simulink model "gm_IP_Core_SS_Switch_and_PWM"  (R2018a)
settings: Solver=VariableStepAuto  StartTime=0.0  StopTime=0.05  RelTol=1e-3
undefined symbols (not defined in the file or in its folder): T_pwm_clk
libraries: hdlmdlgenlib x5, hdlsllib x1
settings Model: Creator=BHK  LastModifiedBy=Wendel
settings OptimizationCC: BlockReduction=off  ConditionallyExecuteInputs=off  DefaultParameterBehavior=Inlined
settings DebuggingCC: AlgebraicLoopMsg=error  InheritedTsInSrcMsg=none
settings HardwareCC: ProdBitPerPointer=32  ProdBitPerSizeT=32  ProdBitPerPtrDiffT=32  ProdLargestAtomicFloat=None  ProdIntDivRoundTo=Undefined  ProdEndianess=Unspecified  ProdWordSize=32  ProdHWDeviceType=ASIC/FPGA->ASIC/FPGA  TargetBitPerPointer=64  TargetBitPerSizeT=64  TargetBitPerPtrDiffT=64  TargetLongLongMode=on  TargetIntDivRoundTo=Zero  TargetEndianess=LittleEndian  TargetWordSize=64  TargetHWDeviceType=Custom Processor->MATLAB Host Computer  ProdEqTarget=off

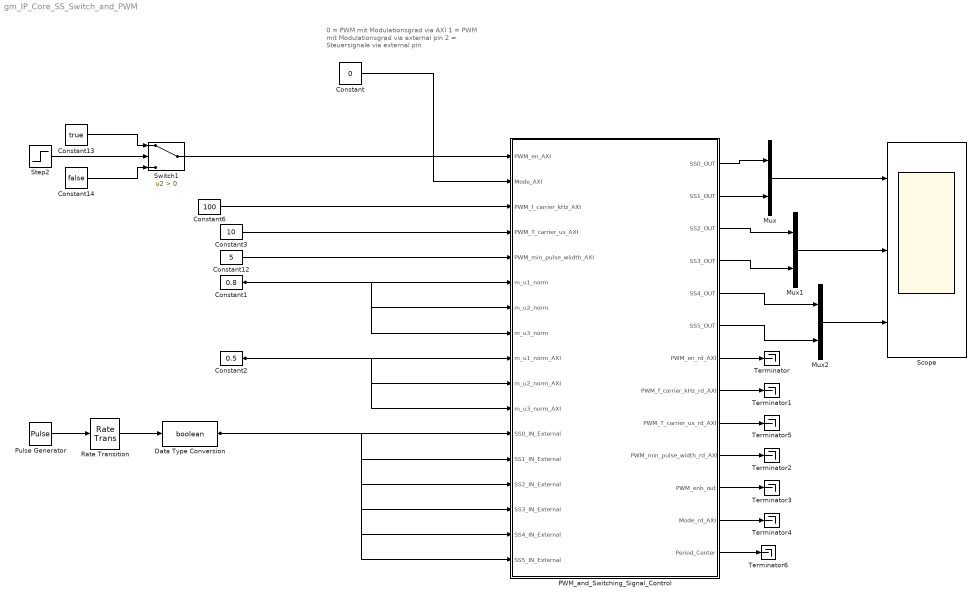
== system gm_IP_Core_SS_Switch_and_PWM ==
  note: 0 = PWM mit Modulationsgrad via AXI
      | 1 = PWM mit Modulationsgrad via external pin
      | 2 = Steuersignale via external pin
  Constant : Constant  Value=0  OutDataTypeStr=fixdt(0,2,0)  SampleTime=T_pwm_clk
  Constant1 : Constant  Value=0.8  OutDataTypeStr=fixdt(1,14,12)  SampleTime=T_pwm_clk
  Constant12 : Constant  Value=5  OutDataTypeStr=fixdt(0,8,0)  SampleTime=T_pwm_clk
  Constant13 : Constant  Value=true  SampleTime=T_pwm_clk
  Constant14 : Constant  Value=false  SampleTime=T_pwm_clk
  Constant2 : Constant  Value=0.5  OutDataTypeStr=fixdt(1,14,12)  SampleTime=T_pwm_clk
  Constant3 : Constant  Value=10  OutDataTypeStr=fixdt(0,8,0)  SampleTime=T_pwm_clk
  Constant6 : Constant  Value=100  OutDataTypeStr=fixdt(0,8,0)  SampleTime=T_pwm_clk
  Data Type Conversion : DataTypeConversion  OutDataTypeStr=boolean
  Mux : Mux  Inputs=2
  Mux1 : Mux  Inputs=2
  Mux2 : Mux  Inputs=2
  PWM_and_Switching_Signal_Control : Subsystem  TreatAsAtomicUnit=on
  Pulse Generator : DiscretePulseGenerator  PulseType=Time based  Period=0.01  PulseWidth=5
  Rate Transition : RateTransition  OutPortSampleTime=T_pwm_clk
  Scope : Scope  NumInputPorts=3
  Step2 : Step  Time=0.002  SampleTime=T_pwm_clk
  Switch1 : Switch  Criteria=u2 > Threshold
  Terminator{,1..6} (7 alike) : Terminator
  wires:
  PWM_and_Switching_Signal_Control/13(Period_Center) -> Terminator6/1
  PWM_and_Switching_Signal_Control/9(PWM_T_carrier_us_rd_AXI) -> Terminator5/1
  Pulse Generator/1 -> Rate Transition/1
  Rate Transition/1 -> Data Type Conversion/1
  Constant3/1 -> PWM_and_Switching_Signal_Control/4(PWM_T_carrier_us_AXI)
  Data Type Conversion/1 -> PWM_and_Switching_Signal_Control/12(SS0_IN_External), PWM_and_Switching_Signal_Control/14(SS2_IN_External), PWM_and_Switching_Signal_Control/16(SS4_IN_External), PWM_and_Switching_Signal_Control/13(SS1_IN_External), PWM_and_Switching_Signal_Control/15(SS3_IN_External), PWM_and_Switching_Signal_Control/17(SS5_IN_External)
  Mux1/1 -> Scope/2
  Mux2/1 -> Scope/3
  PWM_and_Switching_Signal_Control/6(SS5_OUT) -> Mux2/2
  PWM_and_Switching_Signal_Control/5(SS4_OUT) -> Mux2/1
  PWM_and_Switching_Signal_Control/4(SS3_OUT) -> Mux1/2
  PWM_and_Switching_Signal_Control/3(SS2_OUT) -> Mux1/1
  Mux/1 -> Scope/1
  PWM_and_Switching_Signal_Control/2(SS1_OUT) -> Mux/2
  PWM_and_Switching_Signal_Control/1(SS0_OUT) -> Mux/1
  Constant2/1 -> PWM_and_Switching_Signal_Control/11(m_u3_norm_AXI), PWM_and_Switching_Signal_Control/10(m_u2_norm_AXI), PWM_and_Switching_Signal_Control/9(m_u1_norm_AXI)
  PWM_and_Switching_Signal_Control/12(Mode_rd_AXI) -> Terminator4/1
  PWM_and_Switching_Signal_Control/11(PWM_enb_out) -> Terminator3/1
  PWM_and_Switching_Signal_Control/10(PWM_min_pulse_width_rd_AXI) -> Terminator2/1
  PWM_and_Switching_Signal_Control/8(PWM_f_carrier_kHz_rd_AXI) -> Terminator1/1
  PWM_and_Switching_Signal_Control/7(PWM_en_rd_AXI) -> Terminator/1
  Constant1/1 -> PWM_and_Switching_Signal_Control/7(m_u2_norm), PWM_and_Switching_Signal_Control/8(m_u3_norm), PWM_and_Switching_Signal_Control/6(m_u1_norm)
  Constant12/1 -> PWM_and_Switching_Signal_Control/5(PWM_min_pulse_wiidth_AXI)
  Constant6/1 -> PWM_and_Switching_Signal_Control/3(PWM_f_carrier_kHz_AXI)
  Constant/1 -> PWM_and_Switching_Signal_Control/2(Mode_AXI)
  Switch1/1 -> PWM_and_Switching_Signal_Control/1(PWM_en_AXI)
  Constant14/1 -> Switch1/3
  Constant13/1 -> Switch1/1
  Step2/1 -> Switch1/2

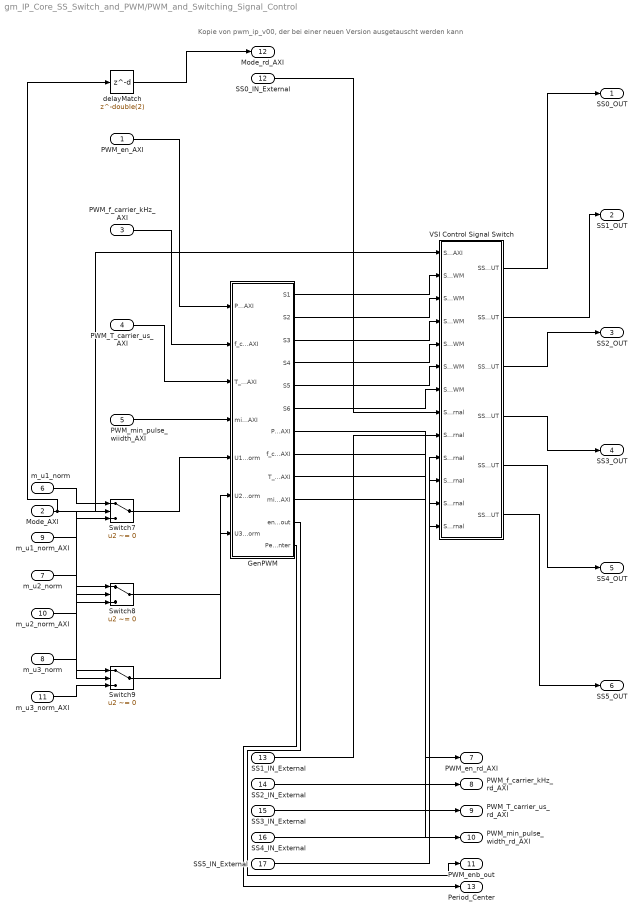
== system gm_IP_Core_SS_Switch_and_PWM/PWM_and_Switching_Signal_Control ==
  note: Kopie von pwm_ip_v00, der bei einer neuen Version ausgetauscht werden kann
  PWM_en_AXI : Inport  OutDataTypeStr=boolean  PortDimensions=1  SampleTime=1e-08
  Mode_AXI : Inport  Port=2  OutDataTypeStr=fixdt(0, 2, 0)  PortDimensions=1  SampleTime=1e-08
  PWM_f_carrier_kHz_AXI : Inport  Port=3  OutDataTypeStr=uint8  PortDimensions=1  SampleTime=1e-08
  PWM_T_carrier_us_AXI : Inport  Port=4  OutDataTypeStr=uint8  PortDimensions=1  SampleTime=1e-08
  PWM_min_pulse_wiidth_AXI : Inport  Port=5  OutDataTypeStr=uint8  PortDimensions=1  SampleTime=1e-08
  m_u1_norm : Inport  Port=6  OutDataTypeStr=fixdt(1, 14, 12)  PortDimensions=1  SampleTime=1e-08
  m_u2_norm : Inport  Port=7  OutDataTypeStr=fixdt(1, 14, 12)  PortDimensions=1  SampleTime=1e-08
  m_u3_norm : Inport  Port=8  OutDataTypeStr=fixdt(1, 14, 12)  PortDimensions=1  SampleTime=1e-08
  m_u1_norm_AXI : Inport  Port=9  OutDataTypeStr=fixdt(1, 14, 12)  PortDimensions=1  SampleTime=1e-08
  m_u2_norm_AXI : Inport  Port=10  OutDataTypeStr=fixdt(1, 14, 12)  PortDimensions=1  SampleTime=1e-08
  m_u3_norm_AXI : Inport  Port=11  OutDataTypeStr=fixdt(1, 14, 12)  PortDimensions=1  SampleTime=1e-08
  SS0_IN_External : Inport  Port=12  OutDataTypeStr=boolean  PortDimensions=1  SampleTime=1e-08
  SS1_IN_External : Inport  Port=13  OutDataTypeStr=boolean  PortDimensions=1  SampleTime=1e-08
  SS2_IN_External : Inport  Port=14  OutDataTypeStr=boolean  PortDimensions=1  SampleTime=1e-08
  SS3_IN_External : Inport  Port=15  OutDataTypeStr=boolean  PortDimensions=1  SampleTime=1e-08
  SS4_IN_External : Inport  Port=16  OutDataTypeStr=boolean  PortDimensions=1  SampleTime=1e-08
  SS5_IN_External : Inport  Port=17  OutDataTypeStr=boolean  PortDimensions=1  SampleTime=1e-08
  GenPWM : Subsystem
  Switch7 : Switch  Criteria=u2 ~= 0  Threshold=double(0)  OutDataTypeStr=fixdt(1, 14, 12)  SampleTime=1e-08
  Switch8 : Switch  Criteria=u2 ~= 0  Threshold=double(0)  OutDataTypeStr=fixdt(1, 14, 12)  SampleTime=1e-08
  Switch9 : Switch  Criteria=u2 ~= 0  Threshold=double(0)  OutDataTypeStr=fixdt(1, 14, 12)  SampleTime=1e-08
  VSI Control Signal Switch : Subsystem
  delayMatch : Delay  DelayLength=double(2)  InitialCondition=0  InputProcessing=Inherited  SampleTime=1e-08
  SS0_OUT : Outport
  SS1_OUT : Outport  Port=2
  SS2_OUT : Outport  Port=3
  SS3_OUT : Outport  Port=4
  SS4_OUT : Outport  Port=5
  SS5_OUT : Outport  Port=6
  PWM_en_rd_AXI : Outport  Port=7
  PWM_f_carrier_kHz_rd_AXI : Outport  Port=8
  PWM_T_carrier_us_rd_AXI : Outport  Port=9
  PWM_min_pulse_width_rd_AXI : Outport  Port=10
  PWM_enb_out : Outport  Port=11
  Mode_rd_AXI : Outport  Port=12
  Period_Center : Outport  Port=13
  wires:
  PWM_en_AXI/1 -> GenPWM/1(PWM_en_AXI)
  delayMatch/1 -> Mode_rd_AXI/1
  PWM_f_carrier_kHz_AXI/1 -> GenPWM/2(f_carrier_kHz_AXI)
  PWM_T_carrier_us_AXI/1 -> GenPWM/3(T_carrier_us_AXI)
  PWM_min_pulse_wiidth_AXI/1 -> GenPWM/4(min_pulse_width_AXI)
  m_u1_norm/1 -> Switch7/1
  m_u2_norm/1 -> Switch8/1
  m_u3_norm/1 -> Switch9/1
  m_u1_norm_AXI/1 -> Switch7/3
  m_u2_norm_AXI/1 -> Switch8/3
  m_u3_norm_AXI/1 -> Switch9/3
  SS0_IN_External/1 -> VSI Control Signal Switch/8(SS0_IN_External)
  SS1_IN_External/1 -> VSI Control Signal Switch/9(SS1_IN_External)
  SS2_IN_External/1 -> VSI Control Signal Switch/10(SS2_IN_External)
  SS3_IN_External/1 -> VSI Control Signal Switch/11(SS3_IN_External)
  SS4_IN_External/1 -> VSI Control Signal Switch/12(SS4_IN_External)
  SS5_IN_External/1 -> VSI Control Signal Switch/13(SS5_IN_External)
  GenPWM/1(S1) -> VSI Control Signal Switch/2(SS0_IN_PWM)
  GenPWM/2(S2) -> VSI Control Signal Switch/3(SS1_IN_PWM)
  GenPWM/3(S3) -> VSI Control Signal Switch/4(SS2_IN_PWM)
  GenPWM/4(S4) -> VSI Control Signal Switch/5(SS3_IN_PWM)
  GenPWM/5(S5) -> VSI Control Signal Switch/6(SS4_IN_PWM)
  GenPWM/6(S6) -> VSI Control Signal Switch/7(SS5_IN_PWM)
  GenPWM/7(PWM_en_rd_AXI) -> PWM_en_rd_AXI/1
  GenPWM/8(f_carrier_kHz_rd_AXI) -> PWM_f_carrier_kHz_rd_AXI/1
  GenPWM/9(T_carrier_us_rd_AXI) -> PWM_T_carrier_us_rd_AXI/1
  GenPWM/10(min_pulse_width_rd_AXI) -> PWM_min_pulse_width_rd_AXI/1
  GenPWM/11(enb_out) -> PWM_enb_out/1
  GenPWM/12(Period_Center) -> Period_Center/1
  Switch7/1 -> GenPWM/5(U1_norm)
  Switch8/1 -> GenPWM/6(U2_norm)
  Switch9/1 -> GenPWM/7(U3_norm)
  VSI Control Signal Switch/1(SS0_OUT) -> SS0_OUT/1
  VSI Control Signal Switch/2(SS1_OUT) -> SS1_OUT/1
  VSI Control Signal Switch/3(SS2_OUT) -> SS2_OUT/1
  VSI Control Signal Switch/4(SS3_OUT) -> SS3_OUT/1
  VSI Control Signal Switch/5(SS4_OUT) -> SS4_OUT/1
  VSI Control Signal Switch/6(SS5_OUT) -> SS5_OUT/1
  Mode_AXI/1 -> delayMatch/1, Switch9/2, Switch8/2, Switch7/2, VSI Control Signal Switch/1(Switch_AXI)

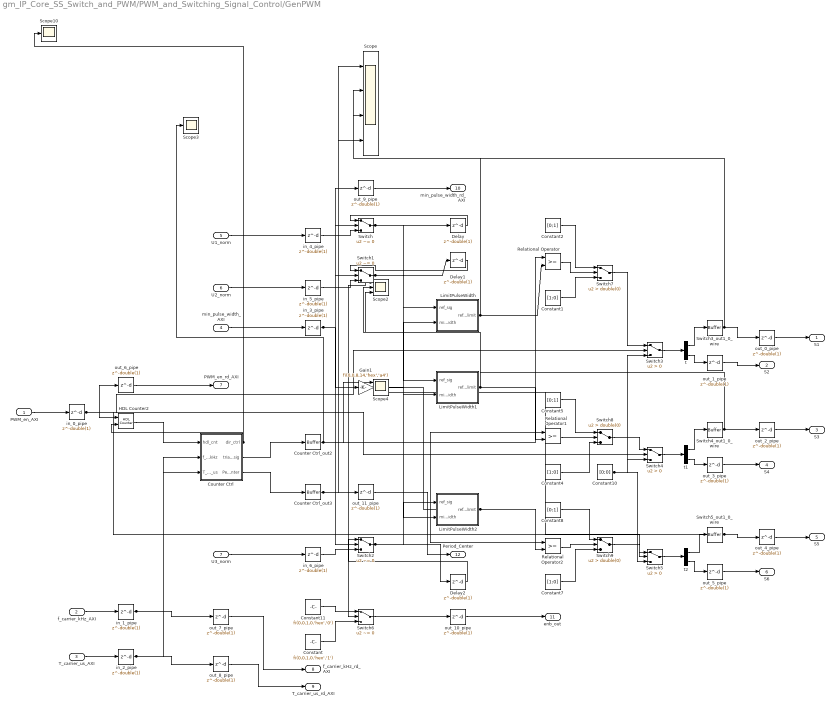
== system gm_IP_Core_SS_Switch_and_PWM/PWM_and_Switching_Signal_Control/GenPWM ==
  PWM_en_AXI : Inport  PortDimensions=1  SampleTime=1e-08
  f_carrier_kHz_AXI : Inport  Port=2  PortDimensions=1  SampleTime=1e-08
  T_carrier_us_AXI : Inport  Port=3  PortDimensions=1  SampleTime=1e-08
  min_pulse_width_AXI : Inport  Port=4  PortDimensions=1  SampleTime=1e-08
  U1_norm : Inport  Port=5  PortDimensions=1  SampleTime=1e-08
  U2_norm : Inport  Port=6  PortDimensions=1  SampleTime=1e-08
  U3_norm : Inport  Port=7  PortDimensions=1  SampleTime=1e-08
  Constant : Constant  Value=fi(0,0,1,0,'hex','1')  OutDataTypeStr=boolean  SampleTime=-1
  Constant1 : Constant  Value=[1;0]  OutDataTypeStr=fixdt(0, 1, 0)  SampleTime=-1
  Constant10 : Constant  Value=[0;0]  OutDataTypeStr=fixdt(0, 1, 0)  SampleTime=-1
  Constant11 : Constant  Value=fi(0,0,1,0,'hex','0')  OutDataTypeStr=boolean  SampleTime=-1
  Constant2 : Constant  Value=[0;1]  OutDataTypeStr=fixdt(0, 1, 0)  SampleTime=-1
  Constant4 : Constant  Value=[1;0]  OutDataTypeStr=fixdt(0, 1, 0)  SampleTime=-1
  Constant5 : Constant  Value=[0;1]  OutDataTypeStr=fixdt(0, 1, 0)  SampleTime=-1
  Constant7 : Constant  Value=[1;0]  OutDataTypeStr=fixdt(0, 1, 0)  SampleTime=-1
  Constant8 : Constant  Value=[0;1]  OutDataTypeStr=fixdt(0, 1, 0)  SampleTime=-1
  Counter Ctrl : Subsystem
  Counter Ctrl_out2 : hdlmdlgenlib/Buffer
      settings: SourceProductName=HDL Coder  SourceProductBaseCode=HD
  Counter Ctrl_out3 : hdlmdlgenlib/Buffer
      settings: SourceProductName=HDL Coder  SourceProductBaseCode=HD
  Delay : Delay  DelayLength=double(1)  InitialCondition=0  InputProcessing=Inherited  SampleTime=1e-08
  Delay1 : Delay  DelayLength=double(1)  InitialCondition=0  InputProcessing=Inherited  SampleTime=1e-08
  Delay2 : Delay  DelayLength=double(1)  InitialCondition=0  InputProcessing=Inherited  SampleTime=1e-08
  Gain1 : Gain  Gain=fi(0,0,8,14,'hex','a4')  ParamDataTypeStr=fixdt(0, 8, 14)  OutDataTypeStr=fixdt(1, 18, 10)  SampleTime=1e-08
  HDL Counter2 : hdlsllib/Sources/HDL Counter  CountType=Free running  CountInit=double(0)  CountStep=double(1)  CountMax=25  CountFromType=Initial value  CountFrom=double(0)  CountResetPort=off  CountLoadPort=off  CountEnbPort=on  CountDirPort=on  CountDataType=Unsigned  CountWordLen=20  CountFracLen=0  CountSampTime=1e-08
      settings: SourceProductBaseCode=HD
  LimitPulseWidth : Subsystem
  LimitPulseWidth1 : Subsystem
  LimitPulseWidth2 : Subsystem
  Relational Operator : RelationalOperator  OutDataTypeStr=boolean  SampleTime=1e-08  RndMeth=Nearest
  Relational Operator1 : RelationalOperator  OutDataTypeStr=boolean  SampleTime=1e-08  RndMeth=Nearest
  Relational Operator2 : RelationalOperator  OutDataTypeStr=boolean  SampleTime=1e-08  RndMeth=Nearest
  Scope : Scope  NumInputPorts=4
  Scope10 : Scope
  Scope2 : Scope  NumInputPorts=3
  Scope3 : Scope
  Scope4 : Scope  NumInputPorts=3
  Switch : Switch  Criteria=u2 ~= 0  Threshold=double(0)  OutDataTypeStr=fixdt(1, 14, 12)  SampleTime=1e-08
  Switch1 : Switch  Criteria=u2 ~= 0  Threshold=double(0)  OutDataTypeStr=fixdt(1, 14, 12)  SampleTime=1e-08
  Switch2 : Switch  Criteria=u2 ~= 0  Threshold=double(0)  OutDataTypeStr=fixdt(1, 14, 12)  SampleTime=1e-08
  Switch3 : Switch  Criteria=u2 > Threshold  OutDataTypeStr=fixdt(0, 1, 0)  SampleTime=1e-08
  Switch3_out1_0_wire : hdlmdlgenlib/Buffer
      settings: SourceProductName=HDL Coder  SourceProductBaseCode=HD
  Switch4 : Switch  Criteria=u2 > Threshold  OutDataTypeStr=fixdt(0, 1, 0)  SampleTime=1e-08
  Switch4_out1_0_wire : hdlmdlgenlib/Buffer
      settings: SourceProductName=HDL Coder  SourceProductBaseCode=HD
  Switch5 : Switch  Criteria=u2 > Threshold  OutDataTypeStr=fixdt(0, 1, 0)  SampleTime=1e-08
  Switch5_out1_0_wire : hdlmdlgenlib/Buffer
      settings: SourceProductName=HDL Coder  SourceProductBaseCode=HD
  Switch6 : Switch  Criteria=u2 ~= 0  Threshold=double(0)  OutDataTypeStr=boolean  SampleTime=1e-08
  Switch7 : Switch  Criteria=u2 > Threshold  Threshold=double(0)  OutDataTypeStr=fixdt(0, 1, 0)  SampleTime=1e-08
  Switch8 : Switch  Criteria=u2 > Threshold  Threshold=double(0)  OutDataTypeStr=fixdt(0, 1, 0)  SampleTime=1e-08
  Switch9 : Switch  Criteria=u2 > Threshold  Threshold=double(0)  OutDataTypeStr=fixdt(0, 1, 0)  SampleTime=1e-08
  in_0_pipe : Delay  DelayLength=double(1)  InitialCondition=0  InputProcessing=Inherited  SampleTime=1e-08
  in_1_pipe : Delay  DelayLength=double(1)  InitialCondition=0  InputProcessing=Inherited  SampleTime=1e-08
  in_2_pipe : Delay  DelayLength=double(1)  InitialCondition=0  InputProcessing=Inherited  SampleTime=1e-08
  in_3_pipe : Delay  DelayLength=double(1)  InitialCondition=0  InputProcessing=Inherited  SampleTime=1e-08
  in_4_pipe : Delay  DelayLength=double(1)  InitialCondition=0  InputProcessing=Inherited  SampleTime=1e-08
  in_5_pipe : Delay  DelayLength=double(1)  InitialCondition=0  InputProcessing=Inherited  SampleTime=1e-08
  in_6_pipe : Delay  DelayLength=double(1)  InitialCondition=0  InputProcessing=Inherited  SampleTime=1e-08
  out_0_pipe : Delay  DelayLength=double(1)  InitialCondition=0  InputProcessing=Inherited  SampleTime=1e-08
  out_10_pipe : Delay  DelayLength=double(1)  InitialCondition=0  InputProcessing=Inherited  SampleTime=1e-08
  out_11_pipe : Delay  DelayLength=double(1)  InitialCondition=0  InputProcessing=Inherited  SampleTime=1e-08
  out_1_pipe : Delay  DelayLength=double(1)  InitialCondition=0  InputProcessing=Inherited  SampleTime=1e-08
  out_2_pipe : Delay  DelayLength=double(1)  InitialCondition=0  InputProcessing=Inherited  SampleTime=1e-08
  out_3_pipe : Delay  DelayLength=double(1)  InitialCondition=0  InputProcessing=Inherited  SampleTime=1e-08
  out_4_pipe : Delay  DelayLength=double(1)  InitialCondition=0  InputProcessing=Inherited  SampleTime=1e-08
  out_5_pipe : Delay  DelayLength=double(1)  InitialCondition=0  InputProcessing=Inherited  SampleTime=1e-08
  out_6_pipe : Delay  DelayLength=double(1)  InitialCondition=0  InputProcessing=Inherited  SampleTime=1e-08
  out_7_pipe : Delay  DelayLength=double(1)  InitialCondition=0  InputProcessing=Inherited  SampleTime=1e-08
  out_8_pipe : Delay  DelayLength=double(1)  InitialCondition=0  InputProcessing=Inherited  SampleTime=1e-08
  out_9_pipe : Delay  DelayLength=double(1)  InitialCondition=0  InputProcessing=Inherited  SampleTime=1e-08
  t : Demux  Outputs=2
  t1 : Demux  Outputs=2
  t2 : Demux  Outputs=2
  S1 : Outport
  S2 : Outport  Port=2
  S3 : Outport  Port=3
  S4 : Outport  Port=4
  S5 : Outport  Port=5
  S6 : Outport  Port=6
  PWM_en_rd_AXI : Outport  Port=7
  f_carrier_kHz_rd_AXI : Outport  Port=8
  T_carrier_us_rd_AXI : Outport  Port=9
  min_pulse_width_rd_AXI : Outport  Port=10
  enb_out : Outport  Port=11
  Period_Center : Outport  Port=12
  wires:
  in_0_pipe/1 -> Switch5/2, Switch4/2, Switch3/2, out_6_pipe/1, HDL Counter2/1
  in_1_pipe/1 -> out_7_pipe/1, Counter Ctrl/2(f_carrier_kHz)
  in_2_pipe/1 -> out_8_pipe/1, Counter Ctrl/3(T_carrier_us)
  in_3_pipe/1 -> out_9_pipe/1, Gain1/1
  in_4_pipe/1 -> Switch/3
  in_5_pipe/1 -> Switch1/3
  in_6_pipe/1 -> Switch2/3
  Constant/1 -> Switch6/3
  Constant1/1 -> Switch7/3
  Constant10/1 -> Switch5/3, Switch4/3, Switch3/3
  Constant11/1 -> Switch6/1
  Constant2/1 -> Switch7/1
  Constant4/1 -> Switch8/3
  Constant5/1 -> Switch8/1
  Constant7/1 -> Switch9/3
  Constant8/1 -> Switch9/1
  Counter Ctrl_out2/1 -> Switch6/2, Relational Operator2/1, Relational Operator1/1, Relational Operator/1, Scope4/1, Scope3/1, Scope2/1, Scope/1, Switch/2, Switch1/2, Switch2/2
  Counter Ctrl_out3/1 -> out_11_pipe/1, Scope/4
  Switch3_out1_0_wire/1 -> out_0_pipe/1, Scope/3
  Switch4_out1_0_wire/1 -> out_2_pipe/1, Scope2/3
  Switch5_out1_0_wire/1 -> out_4_pipe/1, Scope4/3
  Gain1/1 -> LimitPulseWidth/2(min_pulse_width), LimitPulseWidth2/2(min_pulse_width), LimitPulseWidth1/2(min_pulse_width)
  LimitPulseWidth/1(ref_sig_limit) -> Relational Operator/2, Scope/2
  LimitPulseWidth1/1(ref_sig_limit) -> Relational Operator1/2, Scope2/2
  LimitPulseWidth2/1(ref_sig_limit) -> Relational Operator2/2, Scope4/2
  Relational Operator/1 -> Switch7/2
  Relational Operator1/1 -> Switch8/2
  Relational Operator2/1 -> Switch9/2
  Switch3/1 -> t/1
  Switch4/1 -> t1/1
  Switch5/1 -> t2/1
  Switch6/1 -> out_10_pipe/1
  Switch7/1 -> Switch3/1
  Switch8/1 -> Switch4/1
  Switch9/1 -> Switch5/1
  out_0_pipe/1 -> S1/1
  out_1_pipe/1 -> S2/1
  out_2_pipe/1 -> S3/1
  out_3_pipe/1 -> S4/1
  out_4_pipe/1 -> S5/1
  out_5_pipe/1 -> S6/1
  out_6_pipe/1 -> PWM_en_rd_AXI/1
  out_7_pipe/1 -> f_carrier_kHz_rd_AXI/1
  out_8_pipe/1 -> T_carrier_us_rd_AXI/1
  out_9_pipe/1 -> min_pulse_width_rd_AXI/1
  out_10_pipe/1 -> enb_out/1
  out_11_pipe/1 -> Period_Center/1
  t/1 -> Switch3_out1_0_wire/1
  t/2 -> out_1_pipe/1
  t1/1 -> Switch4_out1_0_wire/1
  t1/2 -> out_3_pipe/1
  t2/1 -> Switch5_out1_0_wire/1
  t2/2 -> out_5_pipe/1
  PWM_en_AXI/1 -> in_0_pipe/1
  f_carrier_kHz_AXI/1 -> in_1_pipe/1
  T_carrier_us_AXI/1 -> in_2_pipe/1
  min_pulse_width_AXI/1 -> in_3_pipe/1
  U1_norm/1 -> in_4_pipe/1
  U2_norm/1 -> in_5_pipe/1
  U3_norm/1 -> in_6_pipe/1
  HDL Counter2/1 -> Counter Ctrl/1(hdl_cnt)
  Counter Ctrl/1(dir_ctrl) -> HDL Counter2/2, Scope10/1
  Counter Ctrl/2(triangle_sig) -> Counter Ctrl_out2/1
  Counter Ctrl/3(Period_Center) -> Counter Ctrl_out3/1
  Delay/1 -> Switch/1
  Switch/1 -> Delay/1, LimitPulseWidth/1(ref_sig)
  Delay1/1 -> Switch1/1
  Switch1/1 -> Delay1/1, LimitPulseWidth1/1(ref_sig)
  Delay2/1 -> Switch2/1
  Switch2/1 -> Delay2/1, LimitPulseWidth2/1(ref_sig)

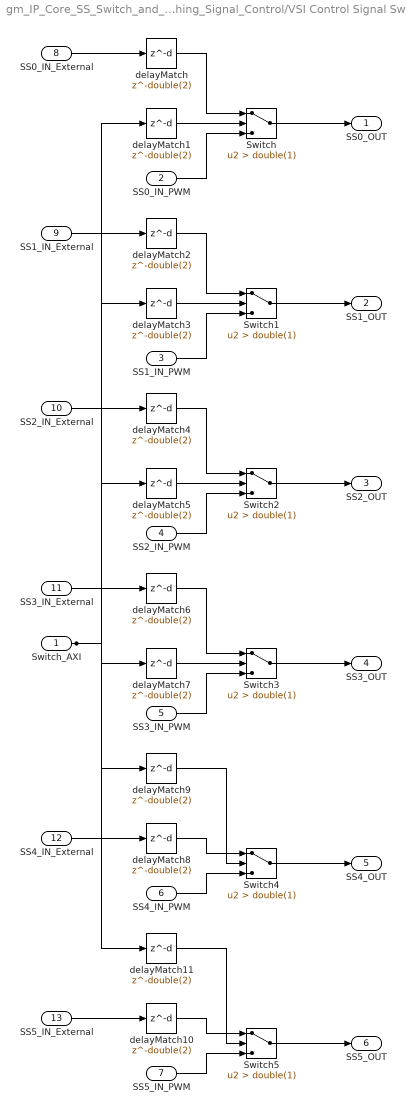
== system gm_IP_Core_SS_Switch_and_PWM/PWM_and_Switching_Signal_Control/VSI Control Signal Switch ==
  Switch_AXI : Inport  PortDimensions=1  SampleTime=1e-08
  SS0_IN_PWM : Inport  Port=2  PortDimensions=1  SampleTime=1e-08
  SS1_IN_PWM : Inport  Port=3  PortDimensions=1  SampleTime=1e-08
  SS2_IN_PWM : Inport  Port=4  PortDimensions=1  SampleTime=1e-08
  SS3_IN_PWM : Inport  Port=5  PortDimensions=1  SampleTime=1e-08
  SS4_IN_PWM : Inport  Port=6  PortDimensions=1  SampleTime=1e-08
  SS5_IN_PWM : Inport  Port=7  PortDimensions=1  SampleTime=1e-08
  SS0_IN_External : Inport  Port=8  PortDimensions=1  SampleTime=1e-08
  SS1_IN_External : Inport  Port=9  PortDimensions=1  SampleTime=1e-08
  SS2_IN_External : Inport  Port=10  PortDimensions=1  SampleTime=1e-08
  SS3_IN_External : Inport  Port=11  PortDimensions=1  SampleTime=1e-08
  SS4_IN_External : Inport  Port=12  PortDimensions=1  SampleTime=1e-08
  SS5_IN_External : Inport  Port=13  PortDimensions=1  SampleTime=1e-08
  Switch{,1..5} (6 alike) : Switch  Criteria=u2 > Threshold  Threshold=double(1)  OutDataTypeStr=boolean  SampleTime=1e-08
  delayMatch{,1..11} (12 alike) : Delay  DelayLength=double(2)  InitialCondition=0  InputProcessing=Inherited  SampleTime=1e-08
  SS0_OUT : Outport
  SS1_OUT : Outport  Port=2
  SS2_OUT : Outport  Port=3
  SS3_OUT : Outport  Port=4
  SS4_OUT : Outport  Port=5
  SS5_OUT : Outport  Port=6
  wires:
  delayMatch1/1 -> Switch/2
  delayMatch/1 -> Switch/1
  delayMatch2/1 -> Switch1/1
  delayMatch4/1 -> Switch2/1
  delayMatch6/1 -> Switch3/1
  delayMatch8/1 -> Switch4/1
  delayMatch10/1 -> Switch5/1
  Switch/1 -> SS0_OUT/1
  Switch1/1 -> SS1_OUT/1
  Switch2/1 -> SS2_OUT/1
  Switch3/1 -> SS3_OUT/1
  Switch4/1 -> SS4_OUT/1
  Switch5/1 -> SS5_OUT/1
  Switch_AXI/1 -> delayMatch11/1, delayMatch9/1, delayMatch7/1, delayMatch5/1, delayMatch3/1, delayMatch1/1
  SS0_IN_PWM/1 -> Switch/3
  SS1_IN_PWM/1 -> Switch1/3
  SS2_IN_PWM/1 -> Switch2/3
  SS3_IN_PWM/1 -> Switch3/3
  SS4_IN_PWM/1 -> Switch4/3
  SS5_IN_PWM/1 -> Switch5/3
  SS0_IN_External/1 -> delayMatch/1
  SS1_IN_External/1 -> delayMatch2/1
  SS2_IN_External/1 -> delayMatch4/1
  SS3_IN_External/1 -> delayMatch6/1
  SS4_IN_External/1 -> delayMatch8/1
  SS5_IN_External/1 -> delayMatch10/1
  delayMatch3/1 -> Switch1/2
  delayMatch5/1 -> Switch2/2
  delayMatch7/1 -> Switch3/2
  delayMatch9/1 -> Switch4/2
  delayMatch11/1 -> Switch5/2

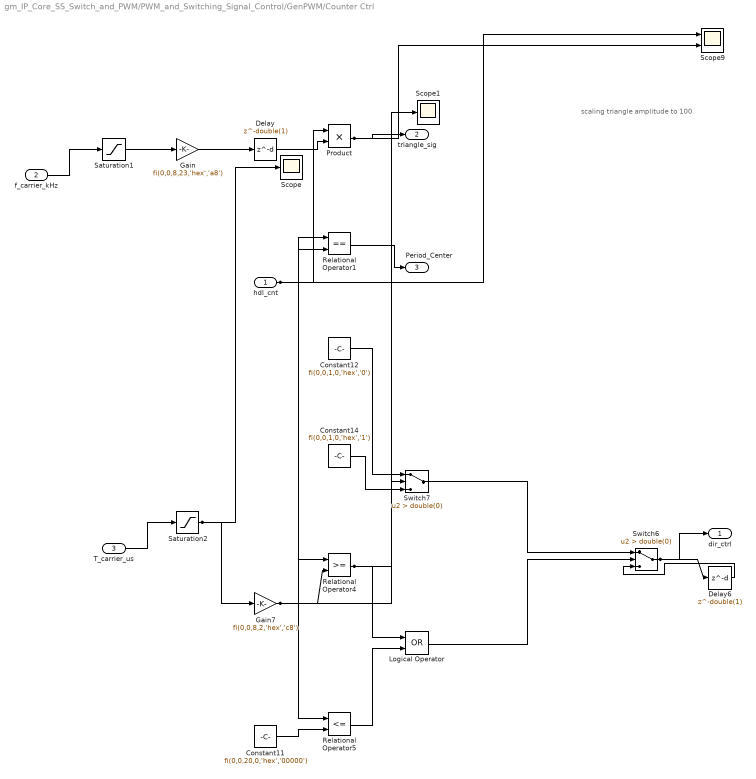
== system gm_IP_Core_SS_Switch_and_PWM/PWM_and_Switching_Signal_Control/GenPWM/Counter Ctrl ==
  note: scaling triangle amplitude to 100
  hdl_cnt : Inport  PortDimensions=1  SampleTime=1e-08
  f_carrier_kHz : Inport  Port=2  PortDimensions=1  SampleTime=1e-08
  T_carrier_us : Inport  Port=3  PortDimensions=1  SampleTime=1e-08
  Constant11 : Constant  Value=fi(0,0,20,0,'hex','00000')  OutDataTypeStr=fixdt(0, 20, 0)  SampleTime=-1
  Constant12 : Constant  Value=fi(0,0,1,0,'hex','0')  OutDataTypeStr=boolean  SampleTime=-1
  Constant14 : Constant  Value=fi(0,0,1,0,'hex','1')  OutDataTypeStr=boolean  SampleTime=-1
  Delay : Delay  DelayLength=double(1)  InitialCondition=0  InputProcessing=Inherited  SampleTime=1e-08
  Delay6 : Delay  DelayLength=double(1)  InitialCondition=0  InputProcessing=Inherited  SampleTime=1e-08
  Gain : Gain  Gain=fi(0,0,8,23,'hex','a8')  ParamDataTypeStr=fixdt(0, 8, 23)  OutDataTypeStr=fixdt(0, 18, 19)  SampleTime=1e-08
  Gain7 : Gain  Gain=fi(0,0,8,2,'hex','c8')  ParamDataTypeStr=fixdt(0, 8, 2)  OutDataTypeStr=fixdt(0, 20, 0)  SampleTime=1e-08
  Logical Operator : Logic  Operator=OR  AllPortsSameDT=off  OutDataTypeStr=boolean  SampleTime=1e-08
  Product : Product  Inputs=**  OutDataTypeStr=fixdt(0, 18, 10)  SampleTime=1e-08
  Relational Operator1 : RelationalOperator  Operator===  OutDataTypeStr=boolean  SampleTime=1e-08  RndMeth=Nearest
  Relational Operator4 : RelationalOperator  OutDataTypeStr=boolean  SampleTime=1e-08  RndMeth=Nearest
  Relational Operator5 : RelationalOperator  Operator=<=  OutDataTypeStr=boolean  SampleTime=1e-08  RndMeth=Nearest
  Saturation1 : Saturate  UpperLimit=fi(0,0,8,0,'hex','64')  LowerLimit=fi(0,0,8,0,'hex','0a')  SampleTime=1e-08  OutDataTypeStr=uint8
  Saturation2 : Saturate  UpperLimit=fi(0,0,8,0,'hex','64')  LowerLimit=fi(0,0,8,0,'hex','0a')  SampleTime=1e-08  OutDataTypeStr=uint8
  Scope : Scope
  Scope1 : Scope
  Scope9 : Scope  NumInputPorts=2
  Switch6 : Switch  Criteria=u2 > Threshold  Threshold=double(0)  OutDataTypeStr=boolean  SampleTime=1e-08
  Switch7 : Switch  Criteria=u2 > Threshold  Threshold=double(0)  OutDataTypeStr=boolean  SampleTime=1e-08
  dir_ctrl : Outport
  triangle_sig : Outport  Port=2
  Period_Center : Outport  Port=3
  wires:
  hdl_cnt/1 -> Relational Operator5/1, Relational Operator4/1, Relational Operator1/1, Product/1, Scope9/1
  f_carrier_kHz/1 -> Saturation1/1
  T_carrier_us/1 -> Saturation2/1
  Constant11/1 -> Relational Operator5/2
  Constant12/1 -> Switch7/1
  Constant14/1 -> Switch7/3
  Delay/1 -> Product/2
  Delay6/1 -> Switch6/3
  Gain/1 -> Delay/1
  Gain7/1 -> Relational Operator4/2, Relational Operator1/2, Scope1/1
  Logical Operator/1 -> Switch6/2
  Product/1 -> Scope9/2, triangle_sig/1
  Relational Operator1/1 -> Period_Center/1
  Relational Operator4/1 -> Switch7/2, Logical Operator/1
  Relational Operator5/1 -> Logical Operator/2
  Saturation1/1 -> Gain/1
  Saturation2/1 -> Scope/1, Gain7/1
  Switch6/1 -> Delay6/1, dir_ctrl/1
  Switch7/1 -> Switch6/1

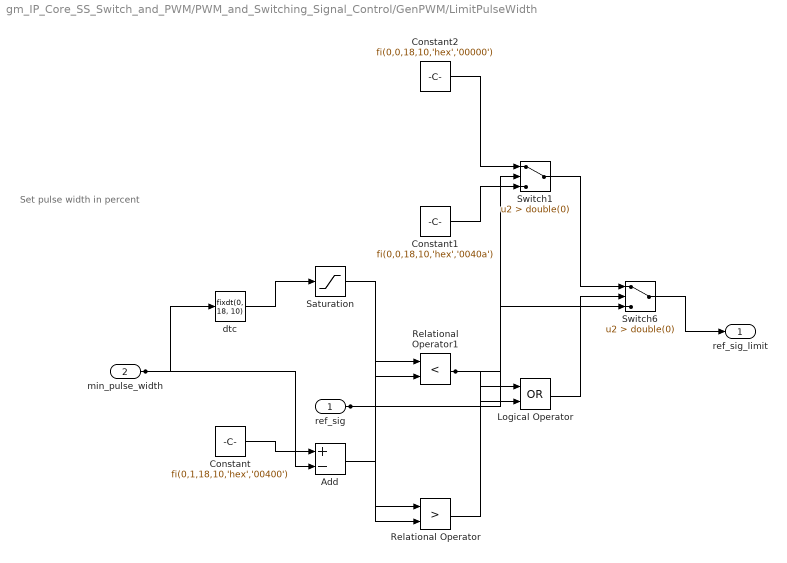
== system gm_IP_Core_SS_Switch_and_PWM/PWM_and_Switching_Signal_Control/GenPWM/LimitPulseWidth ==
  note: Set pulse width in percent
  ref_sig : Inport  PortDimensions=1  SampleTime=1e-08
  min_pulse_width : Inport  Port=2  PortDimensions=1  SampleTime=1e-08
  Add : Sum  Inputs=+-  AccumDataTypeStr=fixdt(1, 19, 10)  OutDataTypeStr=fixdt(0, 18, 10)  SampleTime=1e-08
  Constant : Constant  Value=fi(0,1,18,10,'hex','00400')  OutDataTypeStr=fixdt(1, 18, 10)  SampleTime=-1
  Constant1 : Constant  Value=fi(0,0,18,10,'hex','0040a')  OutDataTypeStr=fixdt(0, 18, 10)  SampleTime=-1
  Constant2 : Constant  Value=fi(0,0,18,10,'hex','00000')  OutDataTypeStr=fixdt(0, 18, 10)  SampleTime=-1
  Logical Operator : Logic  Operator=OR  AllPortsSameDT=off  OutDataTypeStr=boolean  SampleTime=1e-08
  Relational Operator : RelationalOperator  Operator=>  OutDataTypeStr=boolean  SampleTime=1e-08  RndMeth=Nearest
  Relational Operator1 : RelationalOperator  Operator=<  OutDataTypeStr=boolean  SampleTime=1e-08  RndMeth=Nearest
  Saturation : Saturate  UpperLimit=fi(0,0,18,10,'hex','00400')  LowerLimit=fi(0,0,18,10,'hex','00000')  SampleTime=1e-08  OutDataTypeStr=fixdt(0, 18, 10)
  Switch1 : Switch  Criteria=u2 > Threshold  Threshold=double(0)  OutDataTypeStr=fixdt(0, 18, 10)  SampleTime=1e-08
  Switch6 : Switch  Criteria=u2 > Threshold  Threshold=double(0)  OutDataTypeStr=fixdt(0, 18, 10)  SampleTime=1e-08
  dtc : DataTypeConversion  OutDataTypeStr=fixdt(0, 18, 10)  SampleTime=1e-08  SaturateOnIntegerOverflow=on
  ref_sig_limit : Outport
  wires:
  Add/1 -> Relational Operator/2
  Constant/1 -> Add/1
  Constant1/1 -> Switch1/3
  Constant2/1 -> Switch1/1
  Logical Operator/1 -> Switch6/2
  Relational Operator/1 -> Logical Operator/1
  Relational Operator1/1 -> Switch1/2, Logical Operator/2
  Saturation/1 -> Relational Operator1/2
  Switch1/1 -> Switch6/1
  Switch6/1 -> ref_sig_limit/1
  dtc/1 -> Saturation/1
  ref_sig/1 -> Switch6/3, Relational Operator1/1, Relational Operator/1
  min_pulse_width/1 -> dtc/1, Add/2

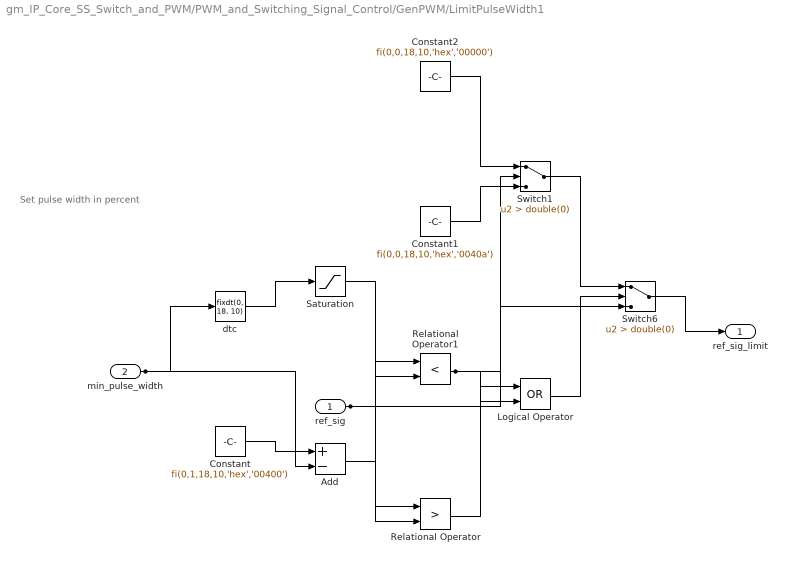
== system gm_IP_Core_SS_Switch_and_PWM/PWM_and_Switching_Signal_Control/GenPWM/LimitPulseWidth1 ==
  note: Set pulse width in percent
  ref_sig : Inport  PortDimensions=1  SampleTime=1e-08
  min_pulse_width : Inport  Port=2  PortDimensions=1  SampleTime=1e-08
  Add : Sum  Inputs=+-  AccumDataTypeStr=fixdt(1, 19, 10)  OutDataTypeStr=fixdt(0, 18, 10)  SampleTime=1e-08
  Constant : Constant  Value=fi(0,1,18,10,'hex','00400')  OutDataTypeStr=fixdt(1, 18, 10)  SampleTime=-1
  Constant1 : Constant  Value=fi(0,0,18,10,'hex','0040a')  OutDataTypeStr=fixdt(0, 18, 10)  SampleTime=-1
  Constant2 : Constant  Value=fi(0,0,18,10,'hex','00000')  OutDataTypeStr=fixdt(0, 18, 10)  SampleTime=-1
  Logical Operator : Logic  Operator=OR  AllPortsSameDT=off  OutDataTypeStr=boolean  SampleTime=1e-08
  Relational Operator : RelationalOperator  Operator=>  OutDataTypeStr=boolean  SampleTime=1e-08  RndMeth=Nearest
  Relational Operator1 : RelationalOperator  Operator=<  OutDataTypeStr=boolean  SampleTime=1e-08  RndMeth=Nearest
  Saturation : Saturate  UpperLimit=fi(0,0,18,10,'hex','00400')  LowerLimit=fi(0,0,18,10,'hex','00000')  SampleTime=1e-08  OutDataTypeStr=fixdt(0, 18, 10)
  Switch1 : Switch  Criteria=u2 > Threshold  Threshold=double(0)  OutDataTypeStr=fixdt(0, 18, 10)  SampleTime=1e-08
  Switch6 : Switch  Criteria=u2 > Threshold  Threshold=double(0)  OutDataTypeStr=fixdt(0, 18, 10)  SampleTime=1e-08
  dtc : DataTypeConversion  OutDataTypeStr=fixdt(0, 18, 10)  SampleTime=1e-08  SaturateOnIntegerOverflow=on
  ref_sig_limit : Outport
  wires:
  Add/1 -> Relational Operator/2
  Constant/1 -> Add/1
  Constant1/1 -> Switch1/3
  Constant2/1 -> Switch1/1
  Logical Operator/1 -> Switch6/2
  Relational Operator/1 -> Logical Operator/1
  Relational Operator1/1 -> Switch1/2, Logical Operator/2
  Saturation/1 -> Relational Operator1/2
  Switch1/1 -> Switch6/1
  Switch6/1 -> ref_sig_limit/1
  dtc/1 -> Saturation/1
  ref_sig/1 -> Switch6/3, Relational Operator1/1, Relational Operator/1
  min_pulse_width/1 -> dtc/1, Add/2

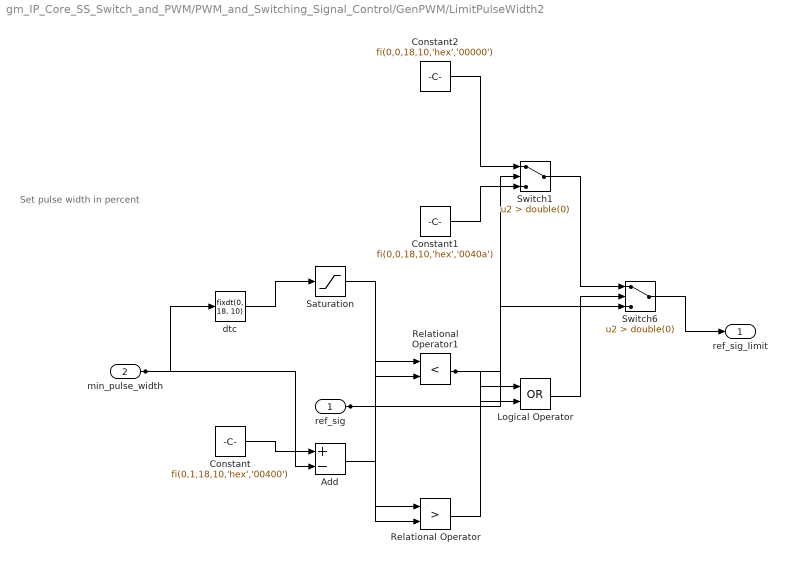
== system gm_IP_Core_SS_Switch_and_PWM/PWM_and_Switching_Signal_Control/GenPWM/LimitPulseWidth2 ==
  note: Set pulse width in percent
  ref_sig : Inport  PortDimensions=1  SampleTime=1e-08
  min_pulse_width : Inport  Port=2  PortDimensions=1  SampleTime=1e-08
  Add : Sum  Inputs=+-  AccumDataTypeStr=fixdt(1, 19, 10)  OutDataTypeStr=fixdt(0, 18, 10)  SampleTime=1e-08
  Constant : Constant  Value=fi(0,1,18,10,'hex','00400')  OutDataTypeStr=fixdt(1, 18, 10)  SampleTime=-1
  Constant1 : Constant  Value=fi(0,0,18,10,'hex','0040a')  OutDataTypeStr=fixdt(0, 18, 10)  SampleTime=-1
  Constant2 : Constant  Value=fi(0,0,18,10,'hex','00000')  OutDataTypeStr=fixdt(0, 18, 10)  SampleTime=-1
  Logical Operator : Logic  Operator=OR  AllPortsSameDT=off  OutDataTypeStr=boolean  SampleTime=1e-08
  Relational Operator : RelationalOperator  Operator=>  OutDataTypeStr=boolean  SampleTime=1e-08  RndMeth=Nearest
  Relational Operator1 : RelationalOperator  Operator=<  OutDataTypeStr=boolean  SampleTime=1e-08  RndMeth=Nearest
  Saturation : Saturate  UpperLimit=fi(0,0,18,10,'hex','00400')  LowerLimit=fi(0,0,18,10,'hex','00000')  SampleTime=1e-08  OutDataTypeStr=fixdt(0, 18, 10)
  Switch1 : Switch  Criteria=u2 > Threshold  Threshold=double(0)  OutDataTypeStr=fixdt(0, 18, 10)  SampleTime=1e-08
  Switch6 : Switch  Criteria=u2 > Threshold  Threshold=double(0)  OutDataTypeStr=fixdt(0, 18, 10)  SampleTime=1e-08
  dtc : DataTypeConversion  OutDataTypeStr=fixdt(0, 18, 10)  SampleTime=1e-08  SaturateOnIntegerOverflow=on
  ref_sig_limit : Outport
  wires:
  Add/1 -> Relational Operator/2
  Constant/1 -> Add/1
  Constant1/1 -> Switch1/3
  Constant2/1 -> Switch1/1
  Logical Operator/1 -> Switch6/2
  Relational Operator/1 -> Logical Operator/1
  Relational Operator1/1 -> Switch1/2, Logical Operator/2
  Saturation/1 -> Relational Operator1/2
  Switch1/1 -> Switch6/1
  Switch6/1 -> ref_sig_limit/1
  dtc/1 -> Saturation/1
  ref_sig/1 -> Switch6/3, Relational Operator1/1, Relational Operator/1
  min_pulse_width/1 -> dtc/1, Add/2
